simulink model "sf_tlevery"  (R2017b)
settings: Solver=ode45  StartTime=0.0  StopTime=100  RelTol=1e-3  EnableMultiTasking=on
settings Model: FPTRunName=Active  ExtModeAutoUpdateStatusClock=off  Creator=The MathWorks, Inc.  LastModifiedBy=The MathWorks, Inc.
settings DataIOCC: LimitDataPoints=on  SaveFormat=Array
settings OptimizationCC: BooleanDataType=off  ExpressionDepthLimit=2147483647  InitFltsAndDblsToZero=on  EfficientMapNaN2IntZero=off  LifeSpan=inf
settings DebuggingCC: SaveWithParameterizedLinksMsg=none  UnderspecifiedInitializationDetection=Classic  MergeDetectMultiDrivingBlocksExec=none  SignalResolutionControl=TryResolveAllWithWarning  MultiTaskDSMMsg=warning  MultiTaskCondExecSysMsg=none  FcnCallInpInsideContextMsg=warning  StateNameClashWarn=warning  StrictBusMsg=None  SFUnexpectedBacktrackingDiag=warning  SFNoUnconditionalDefaultTransitionDiag=warning  SFExecutionAtInitializationDiag=none
settings HardwareCC: ProdBitPerPointer=32  ProdBitPerSizeT=32  ProdBitPerPtrDiffT=32  ProdLargestAtomicFloat=None  ProdIntDivRoundTo=Undefined  ProdEndianess=Unspecified  ProdWordSize=32  ProdHWDeviceType=32-bit Generic  TargetUnknown=on
settings ModelReferenceCC: PropagateSignalLabelsOutOfModel=off
settings SFSimCC: SimParseCustomCode=off
settings CodeAppCC: StateflowObjectComments=on
settings GRTTargetCC: TargetFcnLib=ansi_tfl_tmw.mat  TargetLangStandard=C89/C90 (ANSI)  GeneratePreprocessorConditionals=Disable all  CombineOutputUpdateFcns=off  GRTInterface=on
settings ConfigComp: CovMetricSettings=dcmtr  CovHtmlReporting=on  CovSaveCumulativeToWorkspaceVar=on  CovSaveSingleToWorkspaceVar=on  CovExternalEMLEnable=off  CovSFcnEnable=off

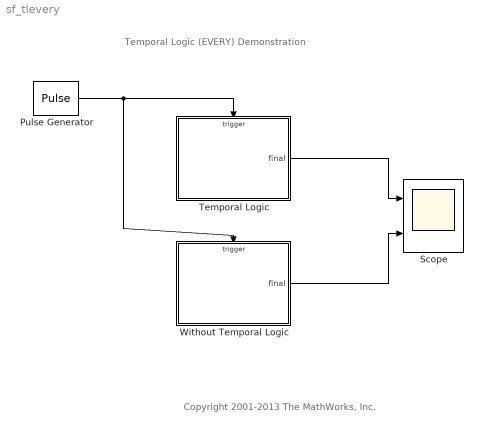
== system sf_tlevery ==
  note: Temporal Logic (EVERY) Demonstration
  note: Copyright 2001-2013 The MathWorks, Inc.
  Pulse Generator : DiscretePulseGenerator  PulseType=Time based  Period=1  PulseWidth=.5
  Scope : Scope  NumInputPorts=2
  Temporal Logic : Stateflow chart  TreatAsAtomicUnit=on
  Without Temporal Logic : Stateflow chart  TreatAsAtomicUnit=on
  wires:
  Pulse Generator/1 -> Temporal Logic/Trigger, Without Temporal Logic/Trigger
  Temporal Logic/1(final) -> Scope/1
  Without Temporal Logic/1(final) -> Scope/2

== stateflow chart sf_tlevery/Without Temporal Logic ==
  state State [parallel]
    settings: executionOrder=1
    state A
    A -> (junction 18) : [count==5]{first_counter = first_counter + 1;}
    (junction 18) -> A : {count=0;}
  state State_two [parallel]
    settings: executionOrder=2
    state B
    B -> (junction 20) : [n==10]{final=double_counter(first_counter);}
    (junction 20) -> B : {n=0;}
  state Counter_two [parallel]
    settings: executionOrder=3
    state Two
      entry: n=1;
      Two -> Two : {n = n + 1;}
  state Counter [parallel]
    settings: executionOrder=4
    state One
      entry: count=1;
      One -> One : {count = count + 1;}
  state output = double_counter(input) [function]
    (default) -> (junction 19) : {output=2.*input;}
  (default) -> A : {first_counter=0;}
  data: input function_input double; output function_output double; count local double; final output double; first_counter local double; n local double
  events: secs input RISING_EDGE_EVENT

== stateflow chart sf_tlevery/Temporal Logic ==
  state Active
    on every(5,secs): count = count + 1;
    on every(10,secs):final=double_counter(count);
  state output = double_counter(input) [function]
    (default) -> (junction 5) : {output=2.*input;}
  (default) -> Active : {count=0;}
  data: input function_input double; output function_output double; count local double; final output double
  events: secs input RISING_EDGE_EVENT
